simulink model "rlSimplePendulumModel2"  (R2023a)
settings: Solver=ode45  StartTime=0.0  StopTime=20  RelTol=1e-5  AbsTol=1e-6
model workspace (MAT data in the model file):
  I = 0
  c = 0
  g = 9.81
  l = 1
  m = 1
  max_tau = 2
  theta0 = 3.14159265359
  theta_dot0 = 0
values from neighbouring files (symbols this model uses):
  mean1 = mean1+k1    (= -0.781844779146)    [calibration.m]    (also in data2.mat = 199.209517856)
  mean2 = mean2+k2    (= -0.473714919647)    [calibration.m]    (also in data2.mat = -0.469851625929)
  std1 = std1*k3    (= 0)    [calibration.m]    (also in data2.mat = 0.432403652579)
  std2 = std2*k4    (= 0)    [calibration.m]    (also in data2.mat = 0.339579901511)
libraries: dspsrcs4 x2, rllib x1
settings Model: Creator=The MathWorks, Inc.  LastModifiedBy=ASKET
settings SolverCC: AutoScaleAbsTol=off  AlgebraicLoopSolver=TrustRegion
settings DataIOCC: LimitDataPoints=on  SaveFormat=Array  SaveState=on
settings OptimizationCC: BlockReduction=off  BooleanDataType=off  LifeSpan=inf
settings DebuggingCC: SaveWithParameterizedLinksMsg=none  SignalResolutionControl=TryResolveAllWithWarning  UnconnectedInputMsg=warning  UnconnectedOutputMsg=warning  UnconnectedLineMsg=warning  SFUnexpectedBacktrackingDiag=warning  SFNoUnconditionalDefaultTransitionDiag=warning  SFExecutionAtInitializationDiag=none  ArithmeticOperatorsInVariantConditions=warning
settings HardwareCC: ProdBitPerPointer=32  ProdBitPerSizeT=32  ProdBitPerPtrDiffT=32  ProdLargestAtomicFloat=None  ProdIntDivRoundTo=Undefined  ProdEndianess=Unspecified  ProdWordSize=32  ProdHWDeviceType=32-bit Generic  TargetUnknown=on
settings ModelReferenceCC: EnableRefExpFcnMdlSchedulingChecks=on  PropagateSignalLabelsOutOfModel=off
settings SFSimCC: SimUseLocalCustomCode=off  CustomCodeUndefinedFunction=UseInterfaceOnly
settings RTWCC: RTWUseLocalCustomCode=off
settings CodeAppCC: StateflowObjectComments=on
settings GRTTargetCC: TargetLangStandard=C89/C90 (ANSI)
settings ConfigComp: CovMetricSettings=dw  CovSaveCumulativeToWorkspaceVar=on  CovSaveSingleToWorkspaceVar=on  CovExternalEMLEnable=off

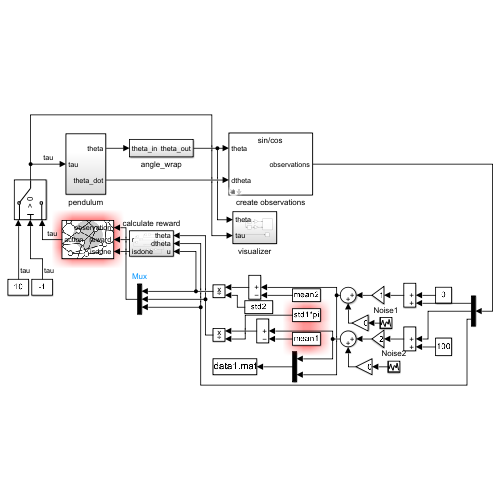
[thumbnail: Simulink's stored preview of the top-level diagram]
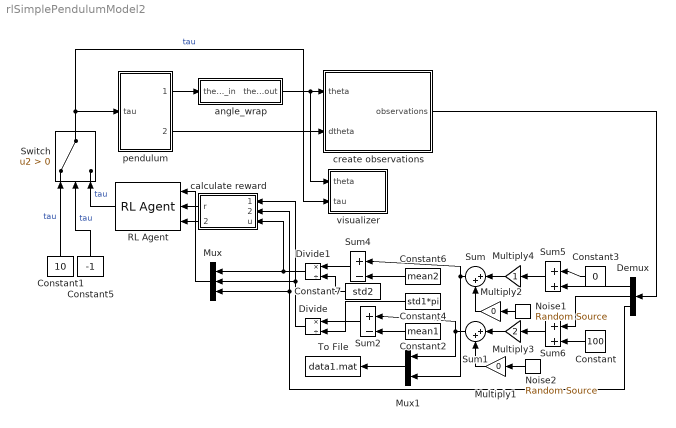
== system rlSimplePendulumModel2 ==
  Constant : Constant  Value=100
  Constant1 : Constant  Value=10
  Constant2 : Constant  Value=mean1
  Constant3 : Constant  Value=0
  Constant4 : Constant  Value=std1*pi
  Constant5 : Constant  Value=-1
  Constant6 : Constant  Value=mean2
  Constant7 : Constant  Value=std2
  Demux : Demux  Outputs=3
  Divide : Product  Inputs=*/
  Divide1 : Product  Inputs=*/
  Multiply1 : Gain  Gain=0
  Multiply2 : Gain  Gain=0
  Multiply3 : Gain  Gain=2
  Multiply4 : Gain
  Mux : Mux  Inputs=3
  Mux1 : Mux  Inputs=2
  Noise1 : dspsrcs4/Random Source  SrcType=Uniform  NormMethod=Sum of uniform values  CltLength=12  MinVal=-0.1  MaxVal=0.1  MeanVal=0  VarVal=1  RepMode=Not repeatable  rawSeed=1  IsInherit=off  SampMode=Continuous  SampTime=0.05  SampFrame=1  DataType=Double  OutComplex=Real  OutputFrames=off
  Noise2 : dspsrcs4/Random Source  SrcType=Uniform  NormMethod=Sum of uniform values  CltLength=12  MinVal=-0.1  MaxVal=0.1  MeanVal=0  VarVal=1  RepMode=Not repeatable  rawSeed=1  IsInherit=off  SampMode=Continuous  SampTime=0.05  SampFrame=1  DataType=Double  OutComplex=Real  OutputFrames=off
  RL Agent : rllib/RL Agent  Agent=agent  ExternalActionAsInput=off  ProvideLastAction=off  ProvideCumRwd=off  TreatAsDirectFeedthrough=on  UseStrictObservationDataTypes=off
  Sum{,1,5..6} (4 alike) : Sum  Inputs=|++
  Sum2 : Sum  Inputs=|+-
  Sum4 : Sum  Inputs=|+-
  Switch : Switch  Criteria=u2 > Threshold  SaturateOnIntegerOverflow=off  InputSameDT=off
  To File : ToFile  Filename=data1.mat  MatrixName=ans1
  angle_wrap : Subsystem
  calculate reward : Subsystem
  create observations : Subsystem  Variant=on  VariantControlMode=label  VariantControl=Variant1  LabelModeActiveChoice=sincos  mask{ThetaObservationHandling=sincos}
      mask prompts: ThetaObservationHandling "Select how theta is treated in the observation vector"
      mask init:
      | simulationStatus = get_param(bdroot,'SimulationStatus');
      | 
      | % The active variant can only be modified at edit-time or very early during
      | % the simulink compile stage. 
      | 
      | choice = get_param(gcb,'ThetaObservationHandling');
      | oldVariant = get_param(gcb,'OverrideUsingVariant');
      | 
      | switch choice
      |     case 'theta'
      |     case 'sincos'
      |     otherwise
      |         error('%s is not supported',choice)
      | end
      | set_param(gcb,'OverrideUsingVariant',choice);
      mask TypeOptions ThetaObservationHandling: theta | sincos
  pendulum : Subsystem
  visualizer : Subsystem
  wires:
  pendulum/1(theta) -> angle_wrap/1(theta_in)
  calculate reward/2(isdone) -> RL Agent/3
  calculate reward/1(r) -> RL Agent/2
  Switch/1 -> pendulum/1(tau), visualizer/2(tau)  "tau"
  create observations/1(" observations") -> Demux/1
  angle_wrap/1(theta_out) -> visualizer/1(theta), create observations/1("theta ")
  pendulum/2(theta_dot) -> create observations/2("dtheta ")
  Constant1/1 -> Switch/1  "tau"
  Constant5/1 -> Switch/2  "tau"
  RL Agent/1 -> Switch/3  "tau"
  Divide/1 -> Mux/2, calculate reward/1(theta)
  Constant4/1 -> Divide/2
  Sum2/1 -> Divide/1
  Sum4/1 -> Divide1/1
  Constant6/1 -> Sum4/2
  Multiply4/1 -> Sum/1
  Noise2/1 -> Multiply1/1
  Multiply1/1 -> Sum1/2
  Multiply2/1 -> Sum/2
  Sum/1 -> Mux1/2, Sum4/1
  Constant2/1 -> Sum2/2
  Noise1/1 -> Multiply2/1
  Sum1/1 -> Sum2/1, Mux1/1
  Sum6/1 -> Multiply3/1
  Mux1/1 -> To File/1
  Multiply3/1 -> Sum1/1
  Constant7/1 -> Divide1/2
  Constant/1 -> Sum6/2
  Sum5/1 -> Multiply4/1
  Demux/2 -> Sum6/1
  Divide1/1 -> Mux/1, calculate reward/3(u)
  Mux/1 -> RL Agent/1
  Demux/3 -> Mux/3, calculate reward/2(dtheta)
  Demux/1 -> Sum5/2
  Constant3/1 -> Sum5/1

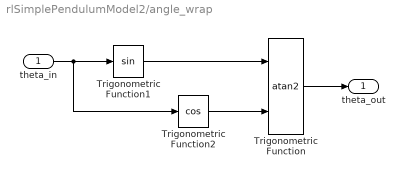
== system rlSimplePendulumModel2/angle_wrap ==
  theta_in : Inport
  Trigonometric Function : Trigonometry  Operator=atan2
  Trigonometric Function1 : Trigonometry
  Trigonometric Function2 : Trigonometry  Operator=cos
  theta_out : Outport  VectorParamsAs1DForOutWhenUnconnected=off
  wires:
  theta_in/1 -> Trigonometric Function2/1, Trigonometric Function1/1
  Trigonometric Function/1 -> theta_out/1
  Trigonometric Function1/1 -> Trigonometric Function/1
  Trigonometric Function2/1 -> Trigonometric Function/2

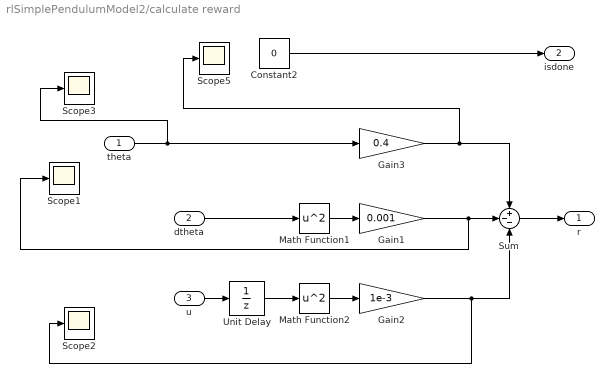
== system rlSimplePendulumModel2/calculate reward ==
  theta : Inport
  dtheta : Inport  Port=2
  u : Inport  Port=3
  Constant2 : Constant  Value=0
  Gain1 : Gain  Gain=0.001
  Gain2 : Gain  Gain=1e-3
  Gain3 : Gain  Gain=0.4
  Math Function1 : Math  Operator=square  SignedPower=on
  Math Function2 : Math  Operator=square  SignedPower=on
  Scope{1..3,5} (4 alike) : Scope
  Sum : Sum  Inputs=+--
  Unit Delay : UnitDelay  SampleTime=-1  HasFrameUpgradeWarning=on
  r : Outport  VectorParamsAs1DForOutWhenUnconnected=off
  isdone : Outport  Port=2  VectorParamsAs1DForOutWhenUnconnected=off
  wires:
  Constant2/1 -> isdone/1
  dtheta/1 -> Math Function1/1
  u/1 -> Unit Delay/1
  Sum/1 -> r/1
  theta/1 -> Gain3/1, Scope3/1
  Math Function1/1 -> Gain1/1
  Math Function2/1 -> Gain2/1
  Gain2/1 -> Scope2/1, Sum/3
  Gain1/1 -> Scope1/1, Sum/2
  Gain3/1 -> Scope5/1, Sum/1
  Unit Delay/1 -> Math Function2/1

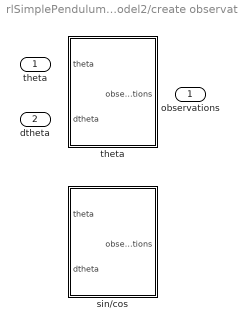
== system rlSimplePendulumModel2/create observations ==
  "theta " : Inport
  "dtheta " : Inport  Port=2
  sin/cos : Subsystem  VariantControl=sincos
  theta : Subsystem  VariantControl=theta
  " observations" : Outport  VectorParamsAs1DForOutWhenUnconnected=off

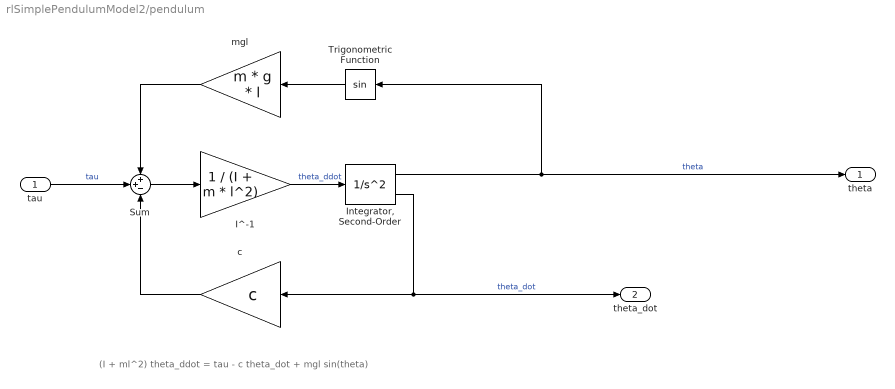
== system rlSimplePendulumModel2/pendulum ==
  note: (I + ml^2) theta_ddot = tau - c theta_dot + mgl sin(theta)
  tau : Inport
  I^-1 : Gain  Gain=1 / (I + m * l^2)
  "Integrator, Second-Order" : SecondOrderIntegrator  ICX=theta0  UpperLimitX=1  LowerLimitX=0  StateNameX='theta'  ICDXDT=theta_dot0  StateNameDXDT='theta_dot'
  Sum : Sum  Inputs=++-
  Trigonometric Function : Trigonometry
  c : Gain  Gain=c
  mgl : Gain  Gain=m * g * l
  theta : Outport  VectorParamsAs1DForOutWhenUnconnected=off
  theta_dot : Outport  Port=2  VectorParamsAs1DForOutWhenUnconnected=off
  wires:
  mgl/1 -> Sum/1
  c/1 -> Sum/3
  Trigonometric Function/1 -> mgl/1
  Sum/1 -> I^-1/1
  "Integrator, Second-Order"/1 -> theta/1, Trigonometric Function/1  "theta"
  I^-1/1 -> "Integrator, Second-Order"/1  "theta_ddot"
  "Integrator, Second-Order"/2 -> c/1, theta_dot/1  "theta_dot"
  tau/1 -> Sum/2  "tau"

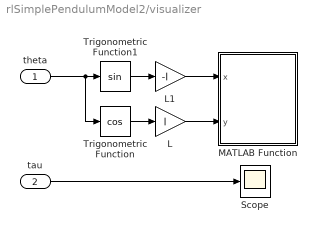
== system rlSimplePendulumModel2/visualizer ==
  theta : Inport
  tau : Inport  Port=2
  L : Gain  Gain=l
  L1 : Gain  Gain=-l
  MATLAB Function : MATLAB Function  TreatAsAtomicUnit=on
  Scope : Scope
  Trigonometric Function : Trigonometry  Operator=cos
  Trigonometric Function1 : Trigonometry
  wires:
  theta/1 -> Trigonometric Function/1, Trigonometric Function1/1
  L1/1 -> MATLAB Function/1(x)
  Trigonometric Function/1 -> L/1
  L/1 -> MATLAB Function/2(y)
  Trigonometric Function1/1 -> L1/1
  tau/1 -> Scope/1

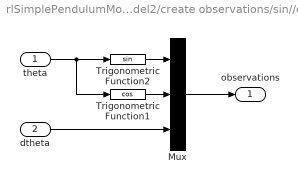
== system rlSimplePendulumModel2/create observations/sin//cos ==
  theta : Inport
  dtheta : Inport  Port=2
  Mux : Mux  Inputs=3
  Trigonometric Function1 : Trigonometry  Operator=cos
  Trigonometric Function2 : Trigonometry
  observations : Outport  VectorParamsAs1DForOutWhenUnconnected=off
  wires:
  theta/1 -> Trigonometric Function1/1, Trigonometric Function2/1
  Mux/1 -> observations/1
  dtheta/1 -> Mux/3
  Trigonometric Function2/1 -> Mux/1
  Trigonometric Function1/1 -> Mux/2

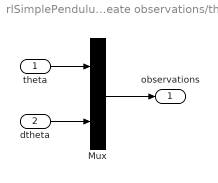
== system rlSimplePendulumModel2/create observations/theta ==
  theta : Inport
  dtheta : Inport  Port=2
  Mux : Mux  Inputs=2
  observations : Outport  VectorParamsAs1DForOutWhenUnconnected=off
  wires:
  dtheta/1 -> Mux/2
  Mux/1 -> observations/1
  theta/1 -> Mux/1

== matlab function rlSimplePendulumModel2/visualizer/MATLAB Function ==
  settings: updateMethod=DISCRETE
  data: x input; y input
function plotPend(x,y)
% plot the simple pendulum
coder.extrinsic('rl.env.viz.plotSimplePendulum');
rl.env.viz.plotSimplePendulum(x,y);
